simulink model "RandomResponseExperiment_Con_Lac"  (R2018a)
settings: Solver=ode5  StartTime=0.0  StopTime=200  FixedStep=Ts  RelTol=1e-3
settings Model: Creator=HTH  LastModifiedBy=DELL
settings OptimizationCC: LifeSpan=inf
settings DebuggingCC: SFExecutionAtInitializationDiag=none
settings CodeAppCC: StateflowObjectComments=on

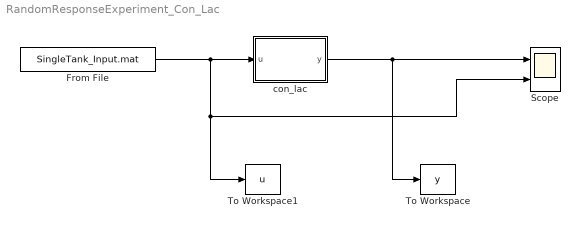
== system RandomResponseExperiment_Con_Lac ==
  From File : FromFile  FileName=SingleTank_Input.mat
  Scope : Scope  NumInputPorts=2
  To Workspace : ToWorkspace  VariableName=y  SampleTime=-1
  To Workspace1 : ToWorkspace  VariableName=u  SampleTime=-1
  con_lac : Subsystem  mask{m=0.3, l=0.5, b=0.2, g=9.81}
  wires:
  From File/1 -> Scope/2, To Workspace1/1, con_lac/1(u)
  con_lac/1(y) -> To Workspace/1, Scope/1

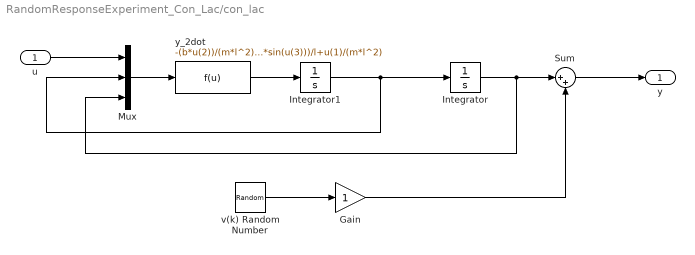
== system RandomResponseExperiment_Con_Lac/con_lac ==
  u : Inport
  Gain : Gain
  Integrator : Integrator  UpperSaturationLimit=pi/3  LowerSaturationLimit=-pi/3
  Integrator1 : Integrator
  Mux : Mux  Inputs=3
  Sum : Sum  Inputs=|++
  v(k) Random Number : RandomNumber  Variance=0.001
  y_2dot : Fcn  Expr=-(b*u(2))/(m*l^2)-(g*sin(u(3)))/l+u(1)/(m*l^2)
  y : Outport
  wires:
  Integrator/1 -> Mux/3, Sum/1
  y_2dot/1 -> Integrator1/1
  Mux/1 -> y_2dot/1
  u/1 -> Mux/1
  Sum/1 -> y/1
  v(k) Random Number/1 -> Gain/1
  Gain/1 -> Sum/2
  Integrator1/1 -> Mux/2, Integrator/1
